simulink model "Decimal"  (R2014a)
settings: Solver=ode45  StartTime=0.0  StopTime=10.0  RelTol=1e-3
libraries: hdlsllib x8
settings Model: Creator=Shiyu  LastModifiedBy=Shiyu

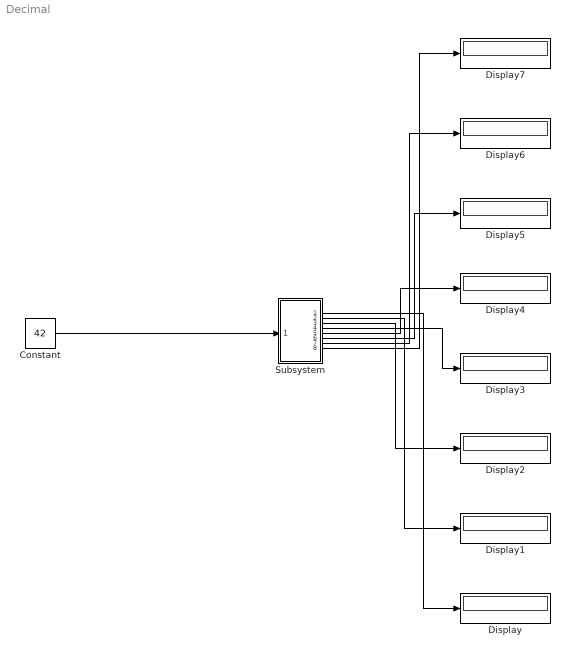
== system Decimal ==
  Constant : Constant  Value=42  OutDataTypeStr=int8
  Display{,1..7} (8 alike) : Display
  Subsystem : Subsystem
  wires:
  Constant/1 -> Subsystem/1(In1)
  Subsystem/1(Out1) -> Display/1
  Subsystem/2(Out2) -> Display1/1
  Subsystem/3(Out3) -> Display2/1
  Subsystem/4(Out4) -> Display3/1
  Subsystem/5(Out5) -> Display4/1
  Subsystem/6(Out6) -> Display5/1
  Subsystem/7(Out7) -> Display6/1
  Subsystem/8(Out8) -> Display7/1

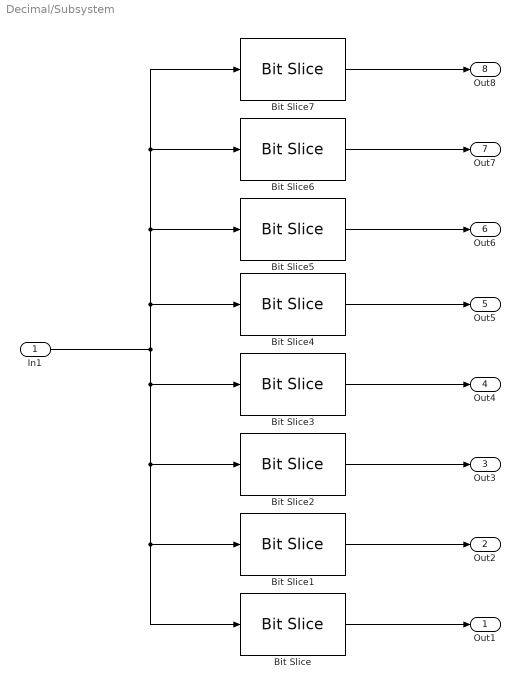
== system Decimal/Subsystem ==
  In1 : Inport  OutDataTypeStr=int8  SampleTime=1
  Bit Slice : hdlsllib/HDL Operations/Bit Slice  lidx=0  ridx=0
  Bit Slice1 : hdlsllib/HDL Operations/Bit Slice  lidx=1  ridx=1
  Bit Slice2 : hdlsllib/HDL Operations/Bit Slice  lidx=2  ridx=2
  Bit Slice3 : hdlsllib/HDL Operations/Bit Slice  lidx=3  ridx=3
  Bit Slice4 : hdlsllib/HDL Operations/Bit Slice  lidx=4  ridx=4
  Bit Slice5 : hdlsllib/HDL Operations/Bit Slice  lidx=5  ridx=5
  Bit Slice6 : hdlsllib/HDL Operations/Bit Slice  lidx=6  ridx=6
  Bit Slice7 : hdlsllib/HDL Operations/Bit Slice  lidx=7  ridx=7
  Out1 : Outport
  Out2 : Outport  Port=2
  Out3 : Outport  Port=3
  Out4 : Outport  Port=4
  Out5 : Outport  Port=5
  Out6 : Outport  Port=6
  Out7 : Outport  Port=7
  Out8 : Outport  Port=8
  wires:
  In1/1 -> Bit Slice7/1, Bit Slice6/1, Bit Slice5/1, Bit Slice4/1, Bit Slice3/1, Bit Slice2/1, Bit Slice1/1, Bit Slice/1
  Bit Slice6/1 -> Out7/1
  Bit Slice3/1 -> Out4/1
  Bit Slice7/1 -> Out8/1
  Bit Slice4/1 -> Out5/1
  Bit Slice1/1 -> Out2/1
  Bit Slice2/1 -> Out3/1
  Bit Slice/1 -> Out1/1
  Bit Slice5/1 -> Out6/1
